simulink model "powersupply"  (R2015b)
settings: Solver=ode45  StartTime=0.0  StopTime=200*T_mach  MaxStep=4e-7  MinStep=1e-8  RelTol=1e-3
values from neighbouring files (symbols this model uses):
  c2_val = (1-V_ref/Vd_val)/(8*v2_ripple*l2_val*f_sw^2)    (= 0.0001)    [PowerSupplyScript.m]    (also in master_conv.m; master_conv2.m; matlab.mat = 1e-05; normal_buck_comparison.m = 1e-05)
  Cs = (Cs_min + Cs_max) / 2    (= 1.43223295455e-05)    [PowerSupplyScript.m]    (also in QdSnubber.m = (Cs_min + Cs_max) / 2; master_conv2.m = 8.70625e-07; matlab.mat = 2.98407954545e-05)
  delay_load = t1    (= 6e-06)    [PowerSupplyScript.m]    (also in master_conv.m; master_conv2.m; matlab.mat)
  delayVC = 2e-3    (= 0.002)    [PowerSupplyScript.m]    (also in master_conv.m = 0.001; master_conv2.m = 0; matlab.mat = 0)
  den_c1 =     [matlab.mat]
  den_c2 =     [matlab.mat]
  duty_inv = 100 - duty    (= 90)    [PowerSupplyScript.m]    (also in master_conv.m; master_conv2.m; matlab.mat)
  duty_load = (t2-t1)/T_mach*100    (= 7)    [PowerSupplyScript.m]    (also in master_conv.m; master_conv2.m; matlab.mat)
  f_sw = 50e3    (= 50000)    [PowerSupplyScript.m]    (also in master_conv.m; master_conv2.m; matlab.mat)
  frq_dc = 10    [master_conv2.m]    (also in matlab.mat)
  I_ref = 10    [PowerSupplyScript.m]    (also in master_conv.m; master_conv2.m; matlab.mat)
  l1_val = Vo1*(Vd_val-Vo1)/(delta_i1*f_sw*Vd_val)    (= 0.00181818181818)    [PowerSupplyScript.m]    (also in master_conv.m = 0.000181818181818; master_conv2.m = 1e-05; matlab.mat; poles_locus.m = l1_val_bak)
  l2_val = 2.5*r_val*(Vd_val-V_ref)/(f_sw*Vd_val)    (= 1.36363636364e-05)    [PowerSupplyScript.m]    (also in master_conv.m; master_conv2.m = 0.0001; matlab.mat = 0.002; poles_locus.m = l2_val_bak)
  num_c1 =     [matlab.mat]
  num_c2 =     [matlab.mat]
  r_val = 1    [PowerSupplyScript.m]    (also in master_conv.m; master_conv2.m; matlab.mat)
  rc2_val = 0.0001    [PowerSupplyScript.m]    (also in master_conv.m; master_conv2.m; matlab.mat)
  rl1_val = 0.0002    [PowerSupplyScript.m]    (also in master_conv.m; master_conv2.m = 0.5; matlab.mat)
  rl2_val = 0.0001    [PowerSupplyScript.m]    (also in master_conv.m; master_conv2.m = 0.1; matlab.mat)
  Rs = V_ref / I_ref    (= 8)    [PowerSupplyScript.m]    (also in QdSnubber.m = V_ref / I_ref; master_conv2.m; matlab.mat)
  t2 = duty * T_mach / 100    (= 2e-05)    [PowerSupplyScript.m]    (also in master_conv.m; master_conv2.m; matlab.mat)
  T_mach = 200e-6    (= 0.0002)    [PowerSupplyScript.m]    (also in master_conv.m; master_conv2.m; matlab.mat)
  V_ref = 80    [PowerSupplyScript.m]    (also in master_conv.m; master_conv2.m; matlab.mat)
  Vd_val = 110    [PowerSupplyScript.m]    (also in master_conv.m; master_conv2.m; matlab.mat)
undefined symbols (not defined in the file or in its folder): dis_den_c1, dis_den_c2, dis_num_c1, dis_num_c2
libraries: powerlib x42, powerlib_meascontrol x7, simulink x3, simulink_extras x2
settings Model: Creator=Akshay  LastModifiedBy=Akshay
settings SolverCC: ZeroCrossAlgorithm=Adaptive
settings DataIOCC: SaveFormat=StructureWithTime
settings HardwareCC: ProdWordSize=32  ProdHWDeviceType=Specified

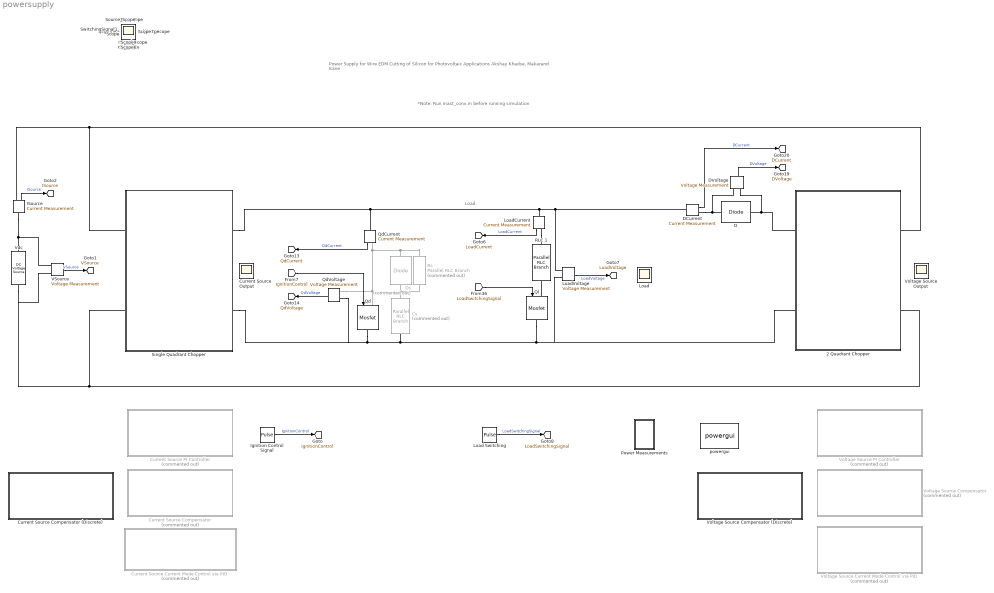
== system powersupply ==
  note: Power Supply for Wire EDM Cutting of Silicon for Photovoltaic Applications
      |
      | Akshay Khadse, Makarand Kane
  note: Load
  note: *Note: Run mast_conv.m before running simulation
  " RLC 1" : powerlib/Elements/Parallel RLC Branch  LConnTagsString=a  RConnTagsString=__new0  BranchType=R  Resistance=r_val  Inductance=1e-3  SetiL0=off  InitialCurrent=0  Capacitance=0.1e-6  Setx0=off  InitialVoltage=0  Measurements=None
  " Rs" : powerlib/Elements/Parallel RLC Branch  Commented=on  LConnTagsString=a  RConnTagsString=__new0  BranchType=R  Resistance=Rs  Inductance=1e-3  SetiL0=off  InitialCurrent=0  Capacitance=0.1e-6  Setx0=off  InitialVoltage=0  Measurements=None
  2 Quadrant Chopper : Subsystem
  Cs : powerlib/Elements/Parallel RLC Branch  Commented=on  LConnTagsString=a  RConnTagsString=__new0  BranchType=C  Resistance=r_val  Inductance=1e-3  SetiL0=off  InitialCurrent=0  Capacitance=Cs  Setx0=off  InitialVoltage=0  Measurements=None
  Current Source Output : Scope
      settings: Floating=on
  Current Source Compensator : Subsystem  Commented=on
  Current Source Compensator (Discrete) : Subsystem
  Current Source Current Mode Control via PID : Subsystem  Commented=on
  Current Source PI Controller : Subsystem  Commented=on
  D : powerlib/Power Electronics/Diode  Ron=0.001  Lon=0  Vf=0.8  IC=0  UseSnubber=off  Rs=1e5  Cs=250e-9  Measurements=off
  DCurrent : powerlib/Measurements/Current Measurement  PhasorSimulation=off  OutputType=Complex  PSBequivalent=0
  DVoltage : powerlib/Measurements/Voltage Measurement  PhasorSimulation=off  OutputType=Complex  PSBequivalent=0
  Ds : powerlib/Power Electronics/Diode  Commented=on  Ron=0.001  Lon=0  Vf=0.8  IC=0  UseSnubber=off  Rs=500  Cs=250e-9  Measurements=off
  ISource : powerlib/Measurements/Current Measurement  PhasorSimulation=off  OutputType=Complex  PSBequivalent=0
  Ignition Control Signal : DiscretePulseGenerator  PulseType=Time based  Period=T_mach  PulseWidth=duty_inv  PhaseDelay=t2 + delayVC
  Load : Scope
      settings: Floating=on
  Load Switching : DiscretePulseGenerator  PulseType=Time based  Period=T_mach  PulseWidth=duty_load  PhaseDelay=delay_load + delayVC
  LoadCurrent : powerlib/Measurements/Current Measurement  PhasorSimulation=off  OutputType=Complex  PSBequivalent=0
  LoadVoltage : powerlib/Measurements/Voltage Measurement  PhasorSimulation=off  OutputType=Complex  PSBequivalent=0
  Power Measurements : Subsystem
  Qd : powerlib/Power Electronics/Mosfet  Ron=0.1  Lon=0  Rd=0.01  Vfd=0  IC=0  Rs=1e5  Cs=inf  Measurements=off
  QdCurrent : powerlib/Measurements/Current Measurement  PhasorSimulation=off  OutputType=Complex  PSBequivalent=0
  QdVoltage : powerlib/Measurements/Voltage Measurement  PhasorSimulation=off  OutputType=Complex  PSBequivalent=0
  Ql : powerlib/Power Electronics/Mosfet  Ron=0.1  Lon=0  Rd=0.01  Vfd=0  IC=0  Rs=1e5  Cs=inf  Measurements=off
  Single Quadrant Chopper : Subsystem
  VSource : powerlib/Measurements/Voltage Measurement  PhasorSimulation=off  OutputType=Complex  PSBequivalent=0
  Vdc : powerlib/Electrical Sources/DC Voltage Source  Amplitude=Vd_val  Measurements=Voltage
  Voltage Source Output : Scope
      settings: Floating=on
  Voltage Source Compensator : Subsystem  Commented=on
  Voltage Source Compensator (Discrete) : Subsystem
  Voltage Source Current Mode Control via PID : Subsystem  Commented=on
  Voltage Source PI Controller : Subsystem  Commented=on
  powergui : powerlib/powergui  Priority=1  SimulationMode=Discrete  SolverType=Backward Euler  SampleTime=0.01/f_sw  frequency=60  SPID=on  DisableSnubberDevices=off  DisableRonSwitches=off  DisableVfSwitches=off  SwTol=0  DisplayEquations=off  Interpol=off  ExternalGateDelay=off  methode=off  Ts=0  FunctionMessages=off  echomessages=off  HookPort=off  EnableUseOfTLC=off  x0status=zero  frequencyindice=0  Pbase=100e6  ErrMax=1e-4  Iterations=50  UnitsV=kV  UnitsW=MW  buscounter=0  RestoreLinks=warning  ResistiveCurrentMeasurement=off  Frange=[0:2:500]  Ylog=off  Xlog=on  ShowGrid=off  save=off  variable=ZData  structure=ScopeData  ZoomFFT=off  StartTime=0.0  cycles=5  DisplayStyle=2  fundamental=50  FreqAxis=off  MaxFrequency=50000  frequencyindicesteady=1  RmsSteady=1  display=off
  C2_Scope : Scope
  D1_Scope : Scope
  D_Scope : Scope
  Ignition_Scope : Scope
  L1_Scope : Scope
  Load_Scope : Scope
  Q1_Scope : Scope
  Q2_Scope : Scope
  Q3_scope : Scope
  Qd_Scope : Scope
  Scope{,1..10} (11 alike) : Scope
  Source_Scope : Scope
  SwitchingSignal1_Scope : Scope
  tag scope: DCurrent=global, DVoltage=global, ISource=global, IgnitionControl=global, LoadCurrent=global, LoadSwitchingSignal=global, LoadVoltage=global, QdCurrent=global, QdVoltage=global, VSource=global
  wires:
  Ignition Control Signal/1 -> [IgnitionControl]  "IgnitionControl"
  Load Switching/1 -> [LoadSwitchingSignal]  "LoadSwitchingSignal"
  LoadCurrent/1 -> [LoadCurrent]  "LoadCurrent"
  LoadVoltage/1 -> [LoadVoltage]  "LoadVoltage"
  [IgnitionControl] -> Qd/1
  QdCurrent/1 -> [QdCurrent]  "QdCurrent"
  QdVoltage/1 -> [QdVoltage]  "QdVoltage"
  DVoltage/1 -> [DVoltage]  "DVoltage"
  DCurrent/1 -> [DCurrent]  "DCurrent"
  [LoadSwitchingSignal] -> Ql/1
  VSource/1 -> [VSource]  "VSource"
  ISource/1 -> [ISource]  "ISource"
  connections:
  LoadCurrent/RConn1 -- " RLC 1"/LConn1
  Ds/LConn1 -- QdVoltage/LConn1 -- Qd/LConn1 -- QdCurrent/RConn1 -- " Rs"/LConn1
  DVoltage/LConn1 -- DCurrent/RConn1 -- D/LConn1
  DCurrent/LConn1 -- LoadVoltage/LConn1 -- LoadCurrent/LConn1 -- Single Quadrant Chopper/RConn1 -- QdCurrent/LConn1
  ISource/RConn1 -- 2 Quadrant Chopper/RConn1 -- Single Quadrant Chopper/LConn1
  VSource/LConn2 -- Vdc/LConn1 -- 2 Quadrant Chopper/RConn2 -- Single Quadrant Chopper/LConn2
  Ql/LConn1 -- " RLC 1"/RConn1
  Qd/RConn1 -- LoadVoltage/LConn2 -- 2 Quadrant Chopper/LConn2 -- Ql/RConn1 -- Cs/RConn1 -- QdVoltage/LConn2 -- Single Quadrant Chopper/RConn2
  ISource/LConn1 -- Vdc/RConn1 -- VSource/LConn1
  Ds/RConn1 -- " Rs"/RConn1 -- Cs/LConn1
  DVoltage/LConn2 -- 2 Quadrant Chopper/LConn1 -- D/RConn1

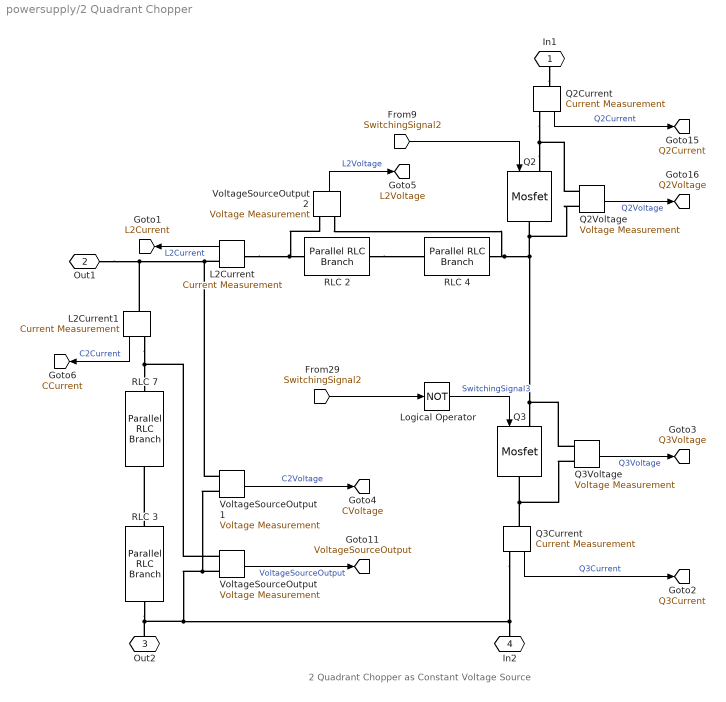
== system powersupply/2 Quadrant Chopper ==
  note: 2 Quadrant Chopper as Constant Voltage Source
  " RLC 2" : powerlib/Elements/Parallel RLC Branch  LConnTagsString=a  RConnTagsString=__new0  BranchType=R  Resistance=rl2_val  Inductance=5e-6  SetiL0=off  InitialCurrent=0  Capacitance=0.3e-6  Setx0=off  InitialVoltage=0  Measurements=None
  " RLC 3" : powerlib/Elements/Parallel RLC Branch  LConnTagsString=a  RConnTagsString=__new0  BranchType=C  Resistance=1  Inductance=1e-3  SetiL0=off  InitialCurrent=0  Capacitance=c2_val  Setx0=off  InitialVoltage=50  Measurements=None
  " RLC 4" : powerlib/Elements/Parallel RLC Branch  LConnTagsString=a  RConnTagsString=__new0  BranchType=L  Resistance=50  Inductance=l2_val  SetiL0=off  InitialCurrent=0  Capacitance=0.3e-6  Setx0=off  InitialVoltage=0  Measurements=None
  " RLC 7" : powerlib/Elements/Parallel RLC Branch  LConnTagsString=a  RConnTagsString=__new0  BranchType=R  Resistance=rc2_val  Inductance=1e-3  SetiL0=off  InitialCurrent=0  Capacitance=0.1e-6  Setx0=off  InitialVoltage=0  Measurements=None
  L2Current : powerlib/Measurements/Current Measurement  PhasorSimulation=off  OutputType=Complex  PSBequivalent=0
  L2Current1 : powerlib/Measurements/Current Measurement  PhasorSimulation=off  OutputType=Complex  PSBequivalent=0
  Logical Operator : Logic  Operator=NOT  AllPortsSameDT=off  OutDataTypeStr=boolean
  Q2 : powerlib/Power Electronics/Mosfet  Ron=0.1  Lon=0  Rd=0.01  Vfd=0  IC=0  Rs=1e5  Cs=inf  Measurements=off
  Q2Current : powerlib/Measurements/Current Measurement  PhasorSimulation=off  OutputType=Complex  PSBequivalent=0
  Q2Voltage : powerlib/Measurements/Voltage Measurement  PhasorSimulation=off  OutputType=Complex  PSBequivalent=0
  Q3 : powerlib/Power Electronics/Mosfet  Ron=0.1  Lon=0  Rd=0.01  Vfd=0  IC=0  Rs=1e5  Cs=inf  Measurements=off
  Q3Current : powerlib/Measurements/Current Measurement  PhasorSimulation=off  OutputType=Complex  PSBequivalent=0
  Q3Voltage : powerlib/Measurements/Voltage Measurement  PhasorSimulation=off  OutputType=Complex  PSBequivalent=0
  VoltageSourceOutput : powerlib/Measurements/Voltage Measurement  PhasorSimulation=off  OutputType=Complex  PSBequivalent=0
  VoltageSourceOutput1 : powerlib/Measurements/Voltage Measurement  PhasorSimulation=off  OutputType=Complex  PSBequivalent=0
  VoltageSourceOutput2 : powerlib/Measurements/Voltage Measurement  PhasorSimulation=off  OutputType=Complex  PSBequivalent=0
  In1 : PMIOPort  Port=1  Side=Right
  Out1 : PMIOPort  Port=2  Side=Left
  Out2 : PMIOPort  Port=3  Side=Left
  In2 : PMIOPort  Port=4  Side=Right
  tag scope: CCurrent=global, CVoltage=global, L2Current=global, L2Voltage=global, Q2Current=global, Q2Voltage=global, Q3Current=global, Q3Voltage=global, VoltageSourceOutput=global
  wires:
  Logical Operator/1 -> Q3/1  "SwitchingSignal3"
  VoltageSourceOutput/1 -> [VoltageSourceOutput]  "VoltageSourceOutput"
  Q3Current/1 -> [Q3Current]  "Q3Current"
  Q3Voltage/1 -> [Q3Voltage]  "Q3Voltage"
  Q2Voltage/1 -> [Q2Voltage]  "Q2Voltage"
  Q2Current/1 -> [Q2Current]  "Q2Current"
  [SwitchingSignal2] -> Q2/1
  [SwitchingSignal2] -> Logical Operator/1
  L2Current/1 -> [L2Current]  "L2Current"
  VoltageSourceOutput1/1 -> [CVoltage]  "C2Voltage"
  VoltageSourceOutput2/1 -> [L2Voltage]  "L2Voltage"
  L2Current1/1 -> [CCurrent]  "C2Current"
  connections:
  " RLC 3"/RConn1 -- In2/RConn1 -- Q3Current/RConn1 -- VoltageSourceOutput1/LConn2 -- VoltageSourceOutput/LConn2 -- Out2/RConn1
  " RLC 3"/LConn1 -- " RLC 7"/RConn1
  Q3Voltage/LConn2 -- Q3Current/LConn1 -- Q3/RConn1
  Q2/LConn1 -- Q2Voltage/LConn1 -- Q2Current/RConn1
  " RLC 2"/RConn1 -- " RLC 4"/LConn1
  In1/RConn1 -- Q2Current/LConn1
  Out1/RConn1 -- VoltageSourceOutput1/LConn1 -- L2Current/RConn1 -- L2Current1/LConn1
  " RLC 4"/RConn1 -- Q3Voltage/LConn1 -- Q3/LConn1 -- Q2Voltage/LConn2 -- Q2/RConn1 -- VoltageSourceOutput2/LConn2
  L2Current/LConn1 -- VoltageSourceOutput2/LConn1 -- " RLC 2"/LConn1
  L2Current1/RConn1 -- VoltageSourceOutput/LConn1 -- " RLC 7"/LConn1

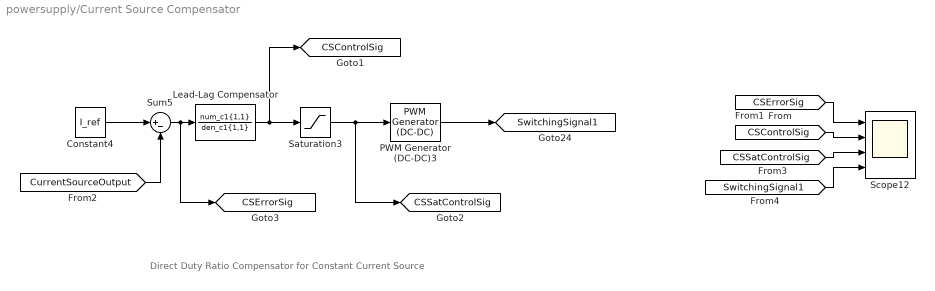
== system powersupply/Current Source Compensator ==
  note: Direct Duty Ratio Compensator for Constant Current Source
  Constant4 : Constant  Value=I_ref
  Lead-Lag Compensator : TransferFcn  Numerator=num_c1{1,1}  Denominator=den_c1{1,1}
  PWM Generator (DC-DC)3 : powerlib_meascontrol/Pulse & Signal Generators/PWM Generator (DC-DC)  Fsw=f_sw  Ts=0
  Saturation3 : Saturate  UpperLimit=0.99  LowerLimit=0
  Scope12 : Scope  NumInputPorts=4
  Sum5 : Sum  Inputs=|+-
  tag scope: CSControlSig=global, CSErrorSig=global, CSSatControlSig=global, SwitchingSignal1=global
  wires:
  Sum5/1 -> [CSErrorSig], Lead-Lag Compensator/1
  Constant4/1 -> Sum5/1
  [CurrentSourceOutput] -> Sum5/2
  Lead-Lag Compensator/1 -> Saturation3/1, [CSControlSig]
  Saturation3/1 -> [CSSatControlSig], PWM Generator (DC-DC)3/1
  PWM Generator (DC-DC)3/1 -> [SwitchingSignal1]
  [CSErrorSig] -> Scope12/1
  [CSControlSig] -> Scope12/2
  [CSSatControlSig] -> Scope12/3
  [SwitchingSignal1] -> Scope12/4

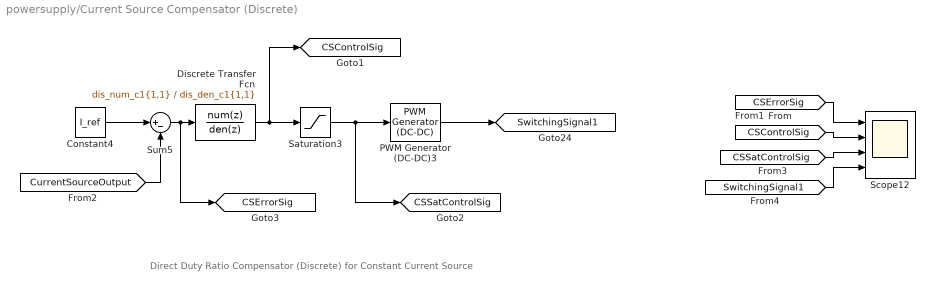
== system powersupply/Current Source Compensator (Discrete) ==
  note: Direct Duty Ratio Compensator (Discrete) for Constant Current Source
  Constant4 : Constant  Value=I_ref
  Discrete Transfer Fcn : DiscreteTransferFcn  Numerator=dis_num_c1{1,1}  Denominator=dis_den_c1{1,1}
  PWM Generator (DC-DC)3 : powerlib_meascontrol/Pulse & Signal Generators/PWM Generator (DC-DC)  Fsw=f_sw  Ts=0
  Saturation3 : Saturate  UpperLimit=0.99  LowerLimit=0
  Scope12 : Scope  NumInputPorts=4
  Sum5 : Sum  Inputs=|+-
  tag scope: CSControlSig=global, CSErrorSig=global, CSSatControlSig=global, SwitchingSignal1=global
  wires:
  Sum5/1 -> Discrete Transfer Fcn/1, [CSErrorSig]
  Constant4/1 -> Sum5/1
  [CurrentSourceOutput] -> Sum5/2
  Discrete Transfer Fcn/1 -> Saturation3/1, [CSControlSig]
  Saturation3/1 -> [CSSatControlSig], PWM Generator (DC-DC)3/1
  PWM Generator (DC-DC)3/1 -> [SwitchingSignal1]
  [CSErrorSig] -> Scope12/1
  [CSControlSig] -> Scope12/2
  [CSSatControlSig] -> Scope12/3
  [SwitchingSignal1] -> Scope12/4

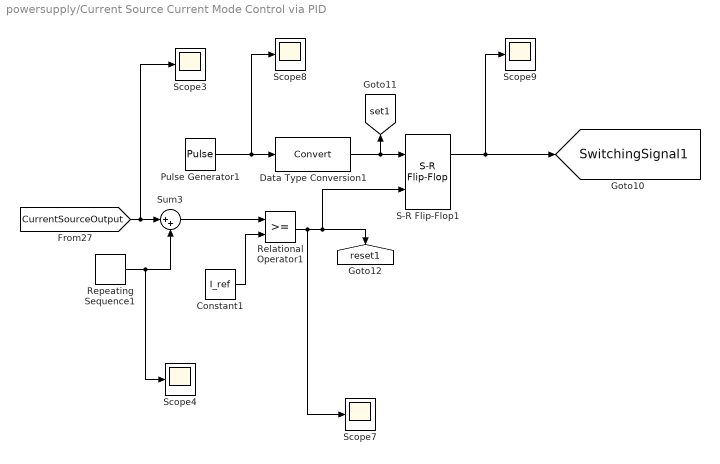
== system powersupply/Current Source Current Mode Control via PID ==
  Constant1 : Constant  Value=I_ref
  Data Type Conversion1 : DataTypeConversion
  Pulse Generator1 : DiscretePulseGenerator  PulseType=Time based  Period=1/f_sw  PulseWidth=5
  Relational Operator1 : RelationalOperator  OutDataTypeStr=boolean
  Repeating Sequence1 : simulink/Sources/Repeating Sequence  rep_seq_t=[0 1/f_sw]  rep_seq_y=[0 0]
  S-R Flip-Flop1 : simulink_extras/Flip Flops/S-R Flip-Flop  initial_condition=0
  Scope{3..4,7..9} (5 alike) : Scope
  Sum3 : Sum  Inputs=|++
  tag scope: SwitchingSignal1=global, reset1=global, set1=global
  wires:
  Pulse Generator1/1 -> Scope8/1, Data Type Conversion1/1
  Data Type Conversion1/1 -> S-R Flip-Flop1/1, [set1]
  Relational Operator1/1 -> Scope7/1, S-R Flip-Flop1/2, [reset1]
  S-R Flip-Flop1/1 -> Scope9/1, [SwitchingSignal1]
  [CurrentSourceOutput] -> Scope3/1, Sum3/1
  Repeating Sequence1/1 -> Scope4/1, Sum3/2
  Sum3/1 -> Relational Operator1/1
  Constant1/1 -> Relational Operator1/2

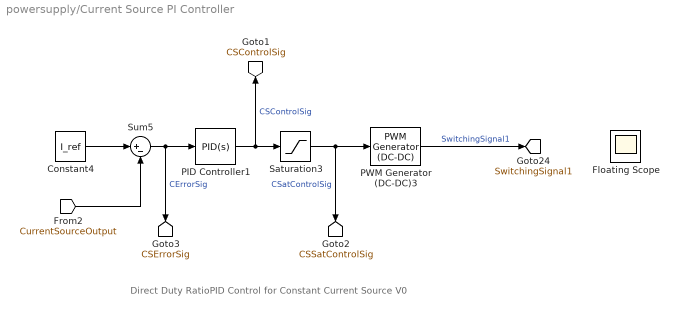
== system powersupply/Current Source PI Controller ==
  note: Direct Duty RatioPID Control for Constant Current Source V0
  Constant4 : Constant  Value=I_ref
  Floating Scope : Scope
      settings: Floating=on
  PID Controller1 : simulink/Continuous/PID Controller  Controller=PID  TimeDomain=Continuous-time  SampleTime=-1  IntegratorMethod=Forward Euler  FilterMethod=Forward Euler  Form=Parallel  UseFilter=on  ControllerParametersSource=internal  P=3  I=0  D=0  N=5  InitialConditionSource=internal  InitialConditionForIntegrator=0  InitialConditionForFilter=0  ExternalReset=none  LimitOutput=off  UpperSaturationLimit=inf  LowerSaturationLimit=-inf  LinearizeAsGain=on  AntiWindupMode=none  Kb=1  TrackingMode=off  Kt=1  PParamMin=[]  PParamMax=[]  IParamMin=[]  IParamMax=[]  DParamMin=[]  DParamMax=[]  NParamMin=[]  NParamMax=[]  KbParamMin=[]  KbParamMax=[]  KtParamMin=[]  KtParamMax=[]  POutMin=[]  POutMax=[]  IOutMin=[]  IOutMax=[]  DOutMin=[]  DOutMax=[]  NOutMin=[]  NOutMax=[]  KbOutMin=[]  KbOutMax=[]  KtOutMin=[]  KtOutMax=[]  IntegratorOutMin=[]  IntegratorOutMax=[]  FilterOutMin=[]  FilterOutMax=[]  SumOutMin=[]  SumOutMax=[]  SumI1OutMin=[]  SumI1OutMax=[]  SumI2OutMin=[]  SumI2OutMax=[]  SumI3OutMin=[]  SumI3OutMax=[]  SumDOutMin=[]  SumDOutMax=[]  SaturationOutMin=[]  SaturationOutMax=[]  IntegratorContinuousStateAttributes=''  IntegratorStateMustResolveToSignalObject=off  IntegratorRTWStateStorageClass=Auto  FilterContinuousStateAttributes=''  FilterStateMustResolveToSignalObject=off  FilterRTWStateStorageClass=Auto  DifferentiatorICPrevScaledInput=0  DifferentiatorOutMin=[]  DifferentiatorOutMax=[]
  PWM Generator (DC-DC)3 : powerlib_meascontrol/Pulse & Signal Generators/PWM Generator (DC-DC)  Fsw=f_sw  Ts=0
  Saturation3 : Saturate  UpperLimit=0.99  LowerLimit=0
  Sum5 : Sum  Inputs=|+-
  tag scope: CSControlSig=global, CSErrorSig=global, CSSatControlSig=global, SwitchingSignal1=global
  wires:
  Sum5/1 -> [CSErrorSig], PID Controller1/1  "CErrorSig"
  Constant4/1 -> Sum5/1
  [CurrentSourceOutput] -> Sum5/2
  PID Controller1/1 -> Saturation3/1, [CSControlSig]  "CSControlSig"
  Saturation3/1 -> [CSSatControlSig], PWM Generator (DC-DC)3/1  "CSatControlSig"
  PWM Generator (DC-DC)3/1 -> [SwitchingSignal1]  "SwitchingSignal1"

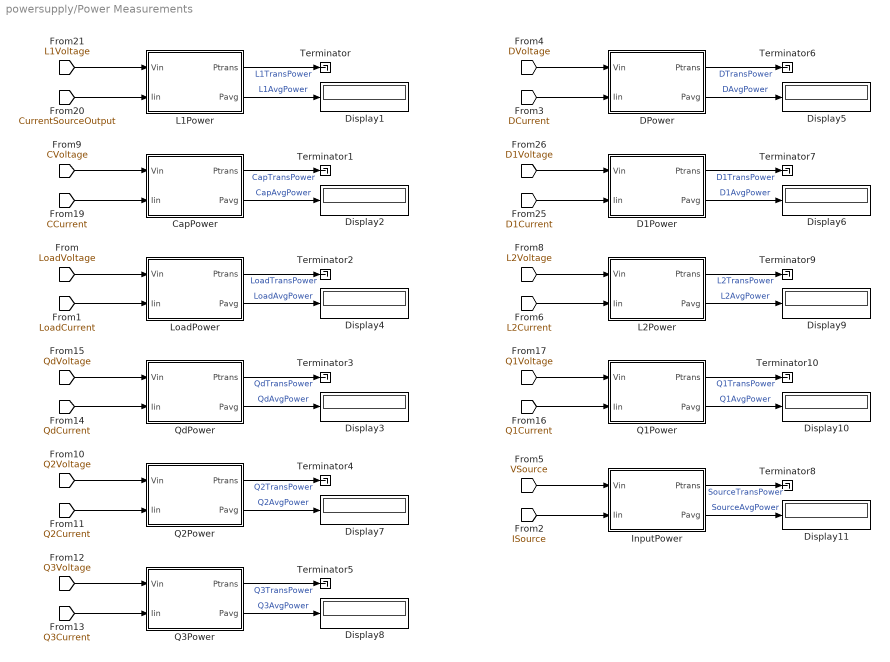
== system powersupply/Power Measurements ==
  CapPower : Subsystem
  D1Power : Subsystem
  DPower : Subsystem
  Display{1..11} (11 alike) : Display
  InputPower : Subsystem
  L1Power : Subsystem
  L2Power : Subsystem
  LoadPower : Subsystem
  Q1Power : Subsystem
  Q2Power : Subsystem
  Q3Power : Subsystem
  QdPower : Subsystem
  Terminator{,1..10} (11 alike) : Terminator
  wires:
  [CVoltage] -> CapPower/1(Vin)
  [CCurrent] -> CapPower/2(Iin)
  CapPower/1(Ptrans) -> Terminator1/1  "CapTransPower"
  CapPower/2(Pavg) -> Display2/1  "CapAvgPower"
  [L1Voltage] -> L1Power/1(Vin)
  [CurrentSourceOutput] -> L1Power/2(Iin)
  L1Power/1(Ptrans) -> Terminator/1  "L1TransPower"
  L1Power/2(Pavg) -> Display1/1  "L1AvgPower"
  [QdVoltage] -> QdPower/1(Vin)
  [QdCurrent] -> QdPower/2(Iin)
  [LoadVoltage] -> LoadPower/1(Vin)
  [LoadCurrent] -> LoadPower/2(Iin)
  LoadPower/1(Ptrans) -> Terminator2/1  "LoadTransPower"
  LoadPower/2(Pavg) -> Display4/1  "LoadAvgPower"
  QdPower/1(Ptrans) -> Terminator3/1  "QdTransPower"
  QdPower/2(Pavg) -> Display3/1  "QdAvgPower"
  [Q2Voltage] -> Q2Power/1(Vin)
  [Q2Current] -> Q2Power/2(Iin)
  [Q3Voltage] -> Q3Power/1(Vin)
  [Q3Current] -> Q3Power/2(Iin)
  Q2Power/1(Ptrans) -> Terminator4/1  "Q2TransPower"
  Q2Power/2(Pavg) -> Display7/1  "Q2AvgPower"
  Q3Power/1(Ptrans) -> Terminator5/1  "Q3TransPower"
  Q3Power/2(Pavg) -> Display8/1  "Q3AvgPower"
  [DVoltage] -> DPower/1(Vin)
  [DCurrent] -> DPower/2(Iin)
  [D1Voltage] -> D1Power/1(Vin)
  [D1Current] -> D1Power/2(Iin)
  DPower/1(Ptrans) -> Terminator6/1  "DTransPower"
  DPower/2(Pavg) -> Display5/1  "DAvgPower"
  D1Power/1(Ptrans) -> Terminator7/1  "D1TransPower"
  D1Power/2(Pavg) -> Display6/1  "D1AvgPower"
  [Q1Voltage] -> Q1Power/1(Vin)
  [Q1Current] -> Q1Power/2(Iin)
  [L2Current] -> L2Power/2(Iin)
  [L2Voltage] -> L2Power/1(Vin)
  Q1Power/2(Pavg) -> Display10/1  "Q1AvgPower"
  Q1Power/1(Ptrans) -> Terminator10/1  "Q1TransPower"
  L2Power/1(Ptrans) -> Terminator9/1  "L2TransPower"
  L2Power/2(Pavg) -> Display9/1  "L2AvgPower"
  [VSource] -> InputPower/1(Vin)
  [ISource] -> InputPower/2(Iin)
  InputPower/1(Ptrans) -> Terminator8/1  "SourceTransPower"
  InputPower/2(Pavg) -> Display11/1  "SourceAvgPower"

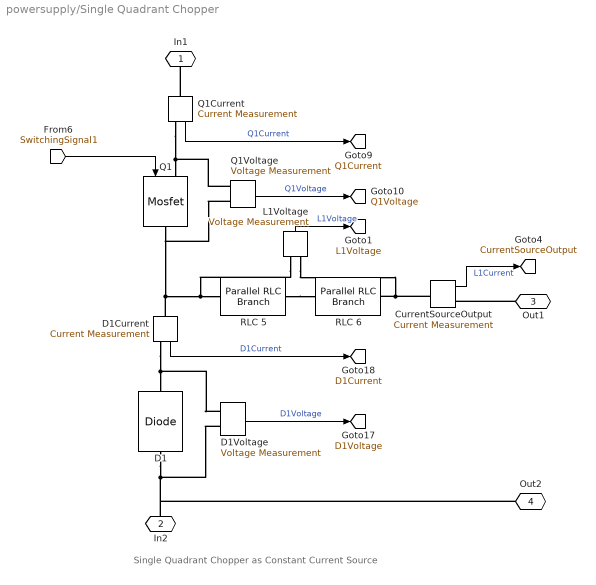
== system powersupply/Single Quadrant Chopper ==
  note: Single Quadrant Chopper as Constant Current Source
  " RLC 5" : powerlib/Elements/Parallel RLC Branch  LConnTagsString=a  RConnTagsString=__new0  BranchType=R  Resistance=rl1_val  Inductance=5e-6  SetiL0=off  InitialCurrent=0  Capacitance=0.3e-6  Setx0=off  InitialVoltage=0  Measurements=None
  " RLC 6" : powerlib/Elements/Parallel RLC Branch  LConnTagsString=a  RConnTagsString=__new0  BranchType=L  Resistance=50  Inductance=l1_val  SetiL0=off  InitialCurrent=100  Capacitance=0.3e-6  Setx0=off  InitialVoltage=0  Measurements=None
  CurrentSourceOutput : powerlib/Measurements/Current Measurement  PhasorSimulation=off  OutputType=Complex  PSBequivalent=0
  D1 : powerlib/Power Electronics/Diode  Ron=0.001  Lon=0  Vf=0.8  IC=0  UseSnubber=off  Rs=1e5  Cs=250e-9  Measurements=off
  D1Current : powerlib/Measurements/Current Measurement  PhasorSimulation=off  OutputType=Complex  PSBequivalent=0
  D1Voltage : powerlib/Measurements/Voltage Measurement  PhasorSimulation=off  OutputType=Complex  PSBequivalent=0
  "L1Voltage " : powerlib/Measurements/Voltage Measurement  PhasorSimulation=off  OutputType=Complex  PSBequivalent=0
  Q1 : powerlib/Power Electronics/Mosfet  Ron=0.1  Lon=0  Rd=0.01  Vfd=0  IC=0  Rs=1e5  Cs=inf  Measurements=off
  Q1Current : powerlib/Measurements/Current Measurement  PhasorSimulation=off  OutputType=Complex  PSBequivalent=0
  Q1Voltage : powerlib/Measurements/Voltage Measurement  PhasorSimulation=off  OutputType=Complex  PSBequivalent=0
  In1 : PMIOPort  Port=1  Side=Left
  In2 : PMIOPort  Port=2  Side=Left
  Out1 : PMIOPort  Port=3  Side=Right
  Out2 : PMIOPort  Port=4  Side=Right
  tag scope: CurrentSourceOutput=global, D1Current=global, D1Voltage=global, L1Voltage=global, Q1Current=global, Q1Voltage=global
  wires:
  CurrentSourceOutput/1 -> [CurrentSourceOutput]  "L1Current"
  [SwitchingSignal1] -> Q1/1
  Q1Current/1 -> [Q1Current]  "Q1Current"
  Q1Voltage/1 -> [Q1Voltage]  "Q1Voltage"
  D1Current/1 -> [D1Current]  "D1Current"
  D1Voltage/1 -> [D1Voltage]  "D1Voltage"
  "L1Voltage "/1 -> [L1Voltage]  "L1Voltage"
  connections:
  Q1Voltage/LConn2 -- Q1/RConn1 -- D1Current/LConn1 -- "L1Voltage "/LConn1 -- " RLC 5"/LConn1
  Q1Current/LConn1 -- In1/RConn1
  " RLC 5"/RConn1 -- " RLC 6"/LConn1
  CurrentSourceOutput/LConn1 -- "L1Voltage "/LConn2 -- " RLC 6"/RConn1
  Q1Current/RConn1 -- Q1Voltage/LConn1 -- Q1/LConn1
  D1Current/RConn1 -- D1/RConn1 -- D1Voltage/LConn1
  D1Voltage/LConn2 -- In2/RConn1 -- Out2/RConn1 -- D1/LConn1
  Out1/RConn1 -- CurrentSourceOutput/RConn1

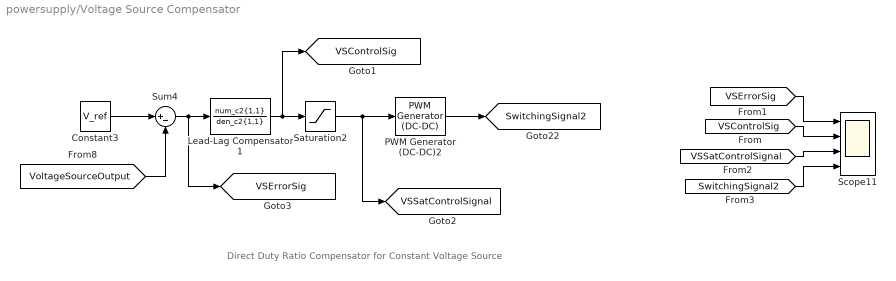
== system powersupply/Voltage Source Compensator ==
  note: Direct Duty Ratio Compensator for Constant Voltage Source
  Constant3 : Constant  Value=V_ref
  Lead-Lag Compensator1 : TransferFcn  Numerator=num_c2{1,1}  Denominator=den_c2{1,1}
  PWM Generator (DC-DC)2 : powerlib_meascontrol/Pulse & Signal Generators/PWM Generator (DC-DC)  Fsw=f_sw  Ts=0
  Saturation2 : Saturate  UpperLimit=0.99  LowerLimit=0
  Scope11 : Scope  NumInputPorts=4
  Sum4 : Sum  Inputs=|+-
  tag scope: SwitchingSignal2=global, VSControlSig=global, VSErrorSig=global, VSSatControlSignal=global
  wires:
  Sum4/1 -> Lead-Lag Compensator1/1, [VSErrorSig]
  Constant3/1 -> Sum4/1
  [VoltageSourceOutput] -> Sum4/2
  Lead-Lag Compensator1/1 -> [VSControlSig], Saturation2/1
  Saturation2/1 -> [VSSatControlSignal], PWM Generator (DC-DC)2/1
  PWM Generator (DC-DC)2/1 -> [SwitchingSignal2]
  [VSErrorSig] -> Scope11/1
  [SwitchingSignal2] -> Scope11/4
  [VSSatControlSignal] -> Scope11/3
  [VSControlSig] -> Scope11/2

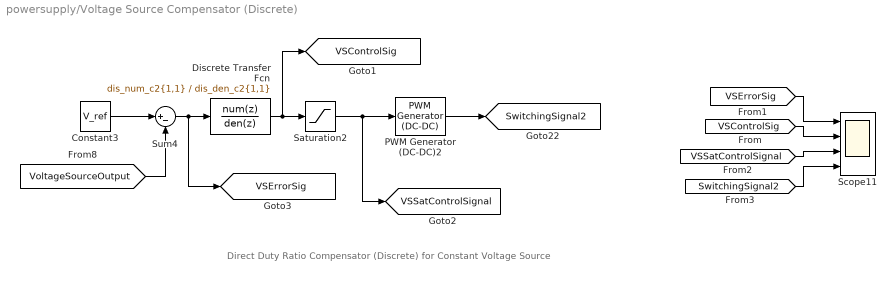
== system powersupply/Voltage Source Compensator (Discrete) ==
  note: Direct Duty Ratio Compensator (Discrete) for Constant Voltage Source
  Constant3 : Constant  Value=V_ref
  Discrete Transfer Fcn : DiscreteTransferFcn  Numerator=dis_num_c2{1,1}  Denominator=dis_den_c2{1,1}
  PWM Generator (DC-DC)2 : powerlib_meascontrol/Pulse & Signal Generators/PWM Generator (DC-DC)  Fsw=f_sw  Ts=0
  Saturation2 : Saturate  UpperLimit=0.99  LowerLimit=0
  Scope11 : Scope  NumInputPorts=4
  Sum4 : Sum  Inputs=|+-
  tag scope: SwitchingSignal2=global, VSControlSig=global, VSErrorSig=global, VSSatControlSignal=global
  wires:
  Sum4/1 -> Discrete Transfer Fcn/1, [VSErrorSig]
  Constant3/1 -> Sum4/1
  [VoltageSourceOutput] -> Sum4/2
  Discrete Transfer Fcn/1 -> [VSControlSig], Saturation2/1
  Saturation2/1 -> [VSSatControlSignal], PWM Generator (DC-DC)2/1
  PWM Generator (DC-DC)2/1 -> [SwitchingSignal2]
  [VSErrorSig] -> Scope11/1
  [SwitchingSignal2] -> Scope11/4
  [VSSatControlSignal] -> Scope11/3
  [VSControlSig] -> Scope11/2

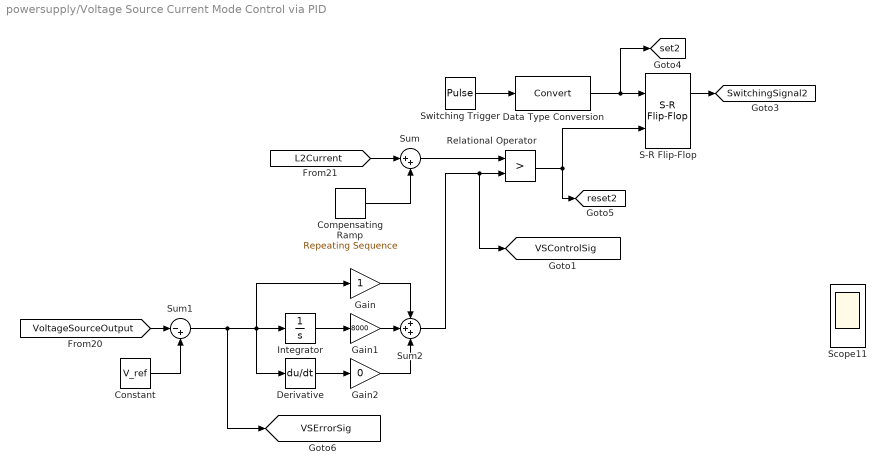
== system powersupply/Voltage Source Current Mode Control via PID ==
  Compensating Ramp : simulink/Sources/Repeating Sequence  rep_seq_t=[0 1/f_sw]  rep_seq_y=[0 80]
  Constant : Constant  Value=V_ref
  Data Type Conversion : DataTypeConversion
  Derivative : Derivative
  Gain : Gain
  Gain1 : Gain  Gain=8000
  Gain2 : Gain  Gain=0
  Integrator : Integrator
  Relational Operator : RelationalOperator  Operator=>  OutDataTypeStr=boolean
  S-R Flip-Flop : simulink_extras/Flip Flops/S-R Flip-Flop  initial_condition=0
  Scope11 : Scope  NumInputPorts=4
  Sum : Sum  Inputs=|++
  Sum1 : Sum  Inputs=|-+
  Sum2 : Sum  Inputs=+++
  Switching Trigger : DiscretePulseGenerator  PulseType=Time based  Period=1/f_sw  PulseWidth=5
  tag scope: SwitchingSignal2=global, VSControlSig=global, VSErrorSig=global, reset2=global, set2=global
  wires:
  Switching Trigger/1 -> Data Type Conversion/1
  Data Type Conversion/1 -> S-R Flip-Flop/1, [set2]
  Relational Operator/1 -> S-R Flip-Flop/2, [reset2]
  S-R Flip-Flop/1 -> [SwitchingSignal2]
  [L2Current] -> Sum/1
  Compensating Ramp/1 -> Sum/2
  Sum/1 -> Relational Operator/1
  [VoltageSourceOutput] -> Sum1/1
  Constant/1 -> Sum1/2
  Sum1/1 -> [VSErrorSig], Derivative/1, Gain/1, Integrator/1
  Integrator/1 -> Gain1/1
  Gain1/1 -> Sum2/2
  Gain/1 -> Sum2/1
  Sum2/1 -> [VSControlSig], Relational Operator/2
  Derivative/1 -> Gain2/1
  Gain2/1 -> Sum2/3

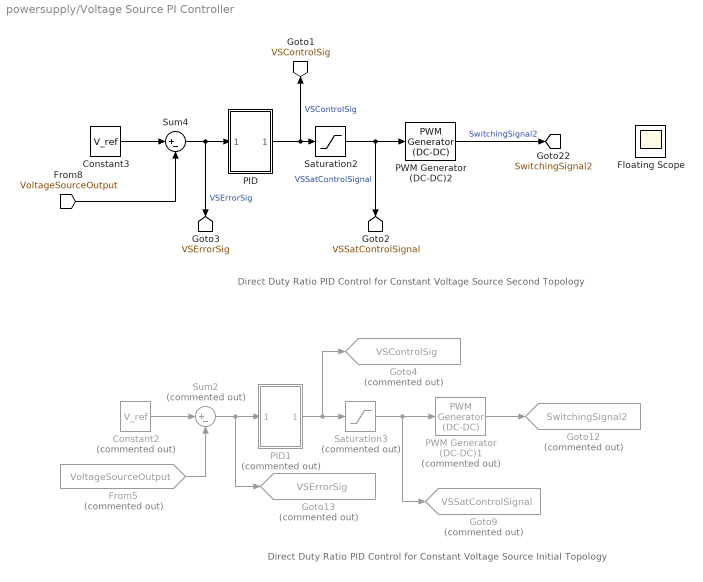
== system powersupply/Voltage Source PI Controller ==
  note: Direct Duty Ratio PID Control for Constant Voltage Source
      | Second Topology
  note: Direct Duty Ratio PID Control for Constant Voltage Source
      | Initial Topology
  Constant2 : Constant  Commented=on  Value=V_ref
  Constant3 : Constant  Value=V_ref
  Floating Scope : Scope
      settings: Floating=on
  From5 : From  Commented=on  GotoTag=VoltageSourceOutput  TagVisibility=global
  Goto12 : Goto  Commented=on  GotoTag=SwitchingSignal2  TagVisibility=global
  Goto13 : Goto  Commented=on  GotoTag=VSErrorSig  TagVisibility=global
  Goto4 : Goto  Commented=on  GotoTag=VSControlSig  TagVisibility=global
  Goto9 : Goto  Commented=on  GotoTag=VSSatControlSignal  TagVisibility=global
  PID : Subsystem
  PID1 : Subsystem  Commented=on
  PWM Generator (DC-DC)1 : powerlib_meascontrol/Pulse & Signal Generators/PWM Generator (DC-DC)  Commented=on  Fsw=f_sw  Ts=0
  PWM Generator (DC-DC)2 : powerlib_meascontrol/Pulse & Signal Generators/PWM Generator (DC-DC)  Fsw=f_sw  Ts=0
  Saturation2 : Saturate  UpperLimit=0.99  LowerLimit=0
  Saturation3 : Saturate  Commented=on  UpperLimit=0.99  LowerLimit=0
  Sum2 : Sum  Commented=on  Inputs=|+-
  Sum4 : Sum  Inputs=|+-
  tag scope: SwitchingSignal2=global, VSControlSig=global, VSErrorSig=global, VSSatControlSignal=global
  wires:
  Constant3/1 -> Sum4/1
  [VoltageSourceOutput] -> Sum4/2
  Saturation2/1 -> [VSSatControlSignal], PWM Generator (DC-DC)2/1  "VSSatControlSignal"
  PWM Generator (DC-DC)2/1 -> [SwitchingSignal2]  "SwitchingSignal2"
  Sum4/1 -> PID/1(In1), [VSErrorSig]  "VSErrorSig"
  PID/1(Out1) -> [VSControlSig], Saturation2/1  "VSControlSig"
  Constant2/1 -> Sum2/1
  From5/1 -> Sum2/2
  Saturation3/1 -> Goto9/1, PWM Generator (DC-DC)1/1
  PWM Generator (DC-DC)1/1 -> Goto12/1
  Sum2/1 -> PID1/1(In1), Goto13/1
  PID1/1(Out1) -> Goto4/1, Saturation3/1

== system powersupply/Power Measurements/CapPower ==
  Vin : Inport
  Iin : Inport  Port=2
  Product : Product
  Transfer Fcn : TransferFcn  Numerator=[2*pi*frq_dc]  Denominator=[1 2*pi*frq_dc]
  Ptrans : Outport
  Pavg : Outport  Port=2
  wires:
  Transfer Fcn/1 -> Pavg/1
  Iin/1 -> Product/2
  Product/1 -> Ptrans/1, Transfer Fcn/1
  Vin/1 -> Product/1

== system powersupply/Power Measurements/D1Power ==
  Vin : Inport
  Iin : Inport  Port=2
  Product : Product
  Transfer Fcn : TransferFcn  Numerator=[2*pi*frq_dc]  Denominator=[1 2*pi*frq_dc]
  Ptrans : Outport
  Pavg : Outport  Port=2
  wires:
  Transfer Fcn/1 -> Pavg/1
  Iin/1 -> Product/2
  Product/1 -> Ptrans/1, Transfer Fcn/1
  Vin/1 -> Product/1

== system powersupply/Power Measurements/DPower ==
  Vin : Inport
  Iin : Inport  Port=2
  Product : Product
  Transfer Fcn : TransferFcn  Numerator=[2*pi*frq_dc]  Denominator=[1 2*pi*frq_dc]
  Ptrans : Outport
  Pavg : Outport  Port=2
  wires:
  Transfer Fcn/1 -> Pavg/1
  Iin/1 -> Product/2
  Product/1 -> Ptrans/1, Transfer Fcn/1
  Vin/1 -> Product/1

== system powersupply/Power Measurements/InputPower ==
  Vin : Inport
  Iin : Inport  Port=2
  Product : Product
  Transfer Fcn : TransferFcn  Numerator=[2*pi*frq_dc]  Denominator=[1 2*pi*frq_dc]
  Ptrans : Outport
  Pavg : Outport  Port=2
  wires:
  Transfer Fcn/1 -> Pavg/1
  Iin/1 -> Product/2
  Product/1 -> Ptrans/1, Transfer Fcn/1
  Vin/1 -> Product/1

== system powersupply/Power Measurements/L1Power ==
  Vin : Inport
  Iin : Inport  Port=2
  Product : Product
  Transfer Fcn : TransferFcn  Numerator=[2*pi*frq_dc]  Denominator=[1 2*pi*frq_dc]
  Ptrans : Outport
  Pavg : Outport  Port=2
  wires:
  Vin/1 -> Product/1
  Product/1 -> Transfer Fcn/1, Ptrans/1
  Iin/1 -> Product/2
  Transfer Fcn/1 -> Pavg/1

== system powersupply/Power Measurements/L2Power ==
  Vin : Inport
  Iin : Inport  Port=2
  Product : Product
  Transfer Fcn : TransferFcn  Numerator=[2*pi*frq_dc]  Denominator=[1 2*pi*frq_dc]
  Ptrans : Outport
  Pavg : Outport  Port=2
  wires:
  Vin/1 -> Product/1
  Product/1 -> Transfer Fcn/1, Ptrans/1
  Iin/1 -> Product/2
  Transfer Fcn/1 -> Pavg/1

== system powersupply/Power Measurements/LoadPower ==
  Vin : Inport
  Iin : Inport  Port=2
  Product : Product
  Transfer Fcn : TransferFcn  Numerator=[2*pi*frq_dc]  Denominator=[1 2*pi*frq_dc]
  Ptrans : Outport
  Pavg : Outport  Port=2
  wires:
  Transfer Fcn/1 -> Pavg/1
  Iin/1 -> Product/2
  Product/1 -> Ptrans/1, Transfer Fcn/1
  Vin/1 -> Product/1

== system powersupply/Power Measurements/Q1Power ==
  Vin : Inport
  Iin : Inport  Port=2
  Product : Product
  Transfer Fcn : TransferFcn  Numerator=[2*pi*frq_dc]  Denominator=[1 2*pi*frq_dc]
  Ptrans : Outport
  Pavg : Outport  Port=2
  wires:
  Vin/1 -> Product/1
  Product/1 -> Transfer Fcn/1, Ptrans/1
  Iin/1 -> Product/2
  Transfer Fcn/1 -> Pavg/1

== system powersupply/Power Measurements/Q2Power ==
  Vin : Inport
  Iin : Inport  Port=2
  Product : Product
  Transfer Fcn : TransferFcn  Numerator=[2*pi*frq_dc]  Denominator=[1 2*pi*frq_dc]
  Ptrans : Outport
  Pavg : Outport  Port=2
  wires:
  Vin/1 -> Product/1
  Product/1 -> Transfer Fcn/1, Ptrans/1
  Iin/1 -> Product/2
  Transfer Fcn/1 -> Pavg/1

== system powersupply/Power Measurements/Q3Power ==
  Vin : Inport
  Iin : Inport  Port=2
  Product : Product
  Transfer Fcn : TransferFcn  Numerator=[2*pi*frq_dc]  Denominator=[1 2*pi*frq_dc]
  Ptrans : Outport
  Pavg : Outport  Port=2
  wires:
  Transfer Fcn/1 -> Pavg/1
  Iin/1 -> Product/2
  Product/1 -> Ptrans/1, Transfer Fcn/1
  Vin/1 -> Product/1

== system powersupply/Power Measurements/QdPower ==
  Vin : Inport
  Iin : Inport  Port=2
  Product : Product
  Transfer Fcn : TransferFcn  Numerator=[2*pi*frq_dc]  Denominator=[1 2*pi*frq_dc]
  Ptrans : Outport
  Pavg : Outport  Port=2
  wires:
  Vin/1 -> Product/1
  Product/1 -> Transfer Fcn/1, Ptrans/1
  Iin/1 -> Product/2
  Transfer Fcn/1 -> Pavg/1

== system powersupply/Voltage Source PI Controller/PID ==
  In1 : Inport
  Derivative : Derivative
  Gain : Gain  Gain=1e6
  Gain1 : Gain  Gain=0
  Gain2 : Gain  Gain=100
  Integrator : Integrator  UpperSaturationLimit=0.99  LowerSaturationLimit=0.01
  Sum : Sum  Inputs=+++
  Out1 : Outport
  wires:
  Gain/1 -> Sum/1
  In1/1 -> Gain1/1, Gain/1, Derivative/1
  Gain2/1 -> Sum/3
  Derivative/1 -> Gain2/1
  Sum/1 -> Out1/1
  Gain1/1 -> Integrator/1
  Integrator/1 -> Sum/2

== system powersupply/Voltage Source PI Controller/PID1 ==
  In1 : Inport
  Derivative : Derivative
  Gain : Gain
  Gain1 : Gain  Gain=60
  Gain2 : Gain  Gain=0
  Integrator : Integrator
  Sum : Sum  Inputs=+++
  Out1 : Outport
  wires:
  Gain/1 -> Sum/1
  In1/1 -> Gain/1, Integrator/1, Derivative/1
  Gain2/1 -> Sum/3
  Gain1/1 -> Sum/2
  Integrator/1 -> Gain1/1
  Derivative/1 -> Gain2/1
  Sum/1 -> Out1/1
